simulink model "lab2"  (R2018a)
settings: Solver=VariableStepAuto  StartTime=0.0  StopTime=2.0  RelTol=1e-3
libraries: simulink x1
settings Model: Creator=Yan Tszyafen  LastModifiedBy=Yan Tszyafen

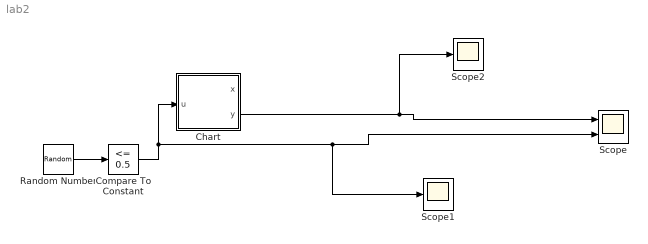
== system lab2 ==
  Chart : Stateflow chart  TreatAsAtomicUnit=on
  Compare To Constant : simulink/Logic and Bit Operations/Compare To Constant  relop=<=  const=0.5  OutDataTypeStr=boolean
  Random Number : RandomNumber  SampleTime=0.1
  Scope : Scope  NumInputPorts=2
  Scope1 : Scope
  Scope2 : Scope
  wires:
  Random Number/1 -> Compare To Constant/1
  Compare To Constant/1 -> Scope1/1, Scope/2, Chart/1(u)
  Chart/2(y) -> Scope2/1, Scope/1

== stateflow chart lab2/Chart ==
  state State1
    x = 0;
  state State2
    x = 1;
  state State3
    x = 2;
  state State4
    x = 3;
  (default) -> State1
  State1 -> State1 [order 1] : [u==0]{y=0;}
  State2 -> State3 [order 1] : [u==0]{y=0;}
  State1 -> State2 [order 2] : [u==1]{y=0;}
  State3 -> State2 [order 2] : [u==1]{y=1;}
  State3 -> State1 [order 1] : [u==0]{y=1;}
  State2 -> State4 [order 2] : [u==1]{y=0;}
  State4 -> State3 [order 1] : [u==0]{y=1;}
  State4 -> State4 [order 2] : [u==1]{y=1;}
  data: u input; x output; y output
